simulink model "steer_by_wire"  (R2019b)
settings: Solver=FixedStepDiscrete  StartTime=0.0  StopTime=inf  RelTol=1e-3  EnableMultiTasking=on
undefined symbols (not defined in the file): DiscIntNeverNeededParam
settings Model: SimulationMode=external  Creator=guest  LastModifiedBy=cernylu6
settings DataIOCC: ReturnWorkspaceOutputs=off
settings OptimizationCC: PassReuseOutputArgsAs=Individual arguments  EfficientTunableParamExpr=on
settings DebuggingCC: ParameterTunabilityLossMsg=error  ArithmeticOperatorsInVariantConditions=warning
settings SFSimCC: SimUseLocalCustomCode=off  MATLABDynamicMemAlloc=off  CustomCodeUndefinedFunction=UseInterfaceOnly
settings RTWCC: Description=Linux Embedded Coder  SystemTargetFile=ert_linux.tlc  MakeCommand="make_rtw OPT_OPTS=\"-O2 -ggdb -Wall\" CC=arm-linux-gnueabihf-gcc CPP=arm-linux-gnueabihf-gcc"  TemplateMakefile=ert_linux.tmf  GenerateReport=on  RTWUseLocalCustomCode=off  IncludeHyperlinkInReport=on  LaunchReport=on  GenerateTraceInfo=on  GenerateTraceReport=on  GenerateTraceReportSl=on  GenerateTraceReportSf=on  GenerateTraceReportEml=on
settings CodeAppCC: ForceParamTrailComments=on  IgnoreCustomStorageClasses=off  OperatorAnnotations=on  SimulinkDataObjDesc=on  SFDataObjDesc=on  MATLABFcnDesc=on  InsertBlockDesc=on  StateflowObjectComments=on  MATLABSourceComments=on
settings STFCustomTargetCC: TargetLangStandard=C99 (ISO)  MultiwordLength=256  ModelReferenceCompliant=off  CombineOutputUpdateFcns=on  ERTCustomFileBanners=on  SupportContinuousTime=off  RemoveResetFunc=on  MATLABClassNameForMDSCustomization=Simulink.SoftwareTarget.ERTCustomization  SystemTargetFile=ert_linux.tlc
settings ERTTargetCC: TargetLangStandard=C99 (ISO)  ModelReferenceCompliant=off  ParMdlRefBuildCompliant=off  CompOptLevelCompliant=off  ConcurrentExecutionCompliant=off  SupportNonInlinedSFcns=on  ModelStepFunctionPrototypeControlCompliant=off  CPPClassGenCompliant=off  UseToolchainInfoCompliant=off  ExtMode=on  ExtModeMexArgs='192.168.136.74'  ERTCustomFileTemplate=ert_linux_file_process.tlc

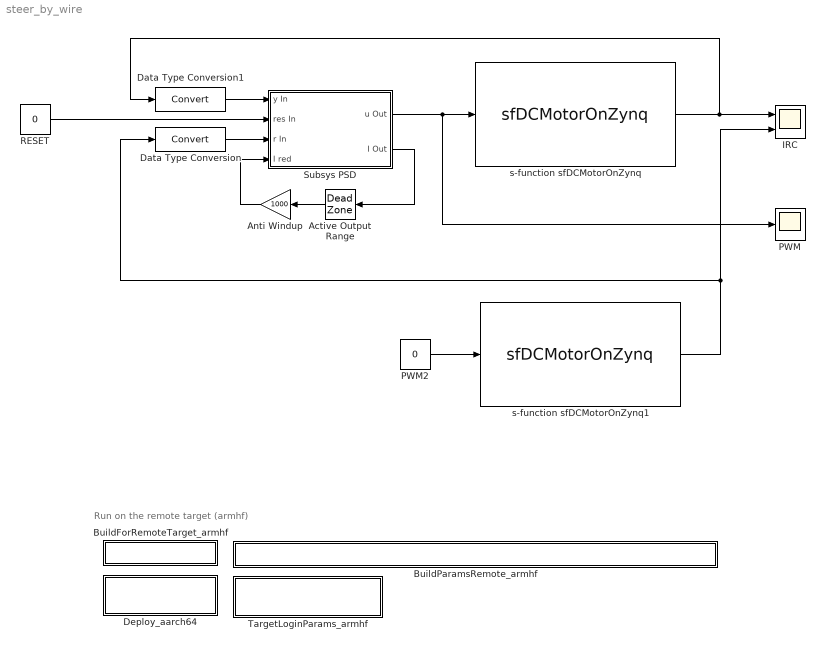
== system steer_by_wire ==
  note: Run on the remote target (armhf)
  "  RESET" : Constant  Value=0
      settings: OpenFcn=if get_param(gcbh,'value')=='0' set_param(gcbh,'value','1'); else set_param(gcbh,'value','0'); end;
  Active Output Range : DeadZone  LowerValue=-1  UpperValue=1  LinearizeAsGain=off
  Anti Windup : Gain  Gain=1000
  BuildForRemoteTarget_armhf : Subsystem
      settings: OpenFcn=ert_linux_build(gcs, 'BuildParamsRemote_armhf')
      mask Display: disp('Build')
  BuildParamsRemote_armhf : Subsystem  mask{make_command='make_rtw OPT_OPTS="-O2 -ggdb -Wall" CC=arm-linux-gnueabihf-gcc CPP=arm-linux-gnueabihf-gcc'}
      mask prompts: make_command "MakeCommand"
      mask Display: disp(get_param(gcb, 'make_command'));
  Data Type Conversion : DataTypeConversion
  Data Type Conversion1 : DataTypeConversion
  Deploy_aarch64 : Subsystem
      settings: OpenFcn=ert_linux_deploy_and_connect(gcs, 'TargetLoginParams_armhf');
      mask Display: disp('Deploy and\nconnect')
  IRC : Scope  NumInputPorts=2
  PWM : Scope
  PWM2 : Constant  Value=0
  Subsys PSD : Subsystem  mask(optimized PSD controller){P=0.01, I=0.1, D=0.0001, Ts=0.001}
      mask prompts: P "P proportional (P):"; I "I integral (I):"; D "D derivative (D):"; Ts "Sampling period (Ts):"
      mask help:
      | Type: Subsystem block.
      |
      | Description:
      |   Subsystem covers optimized PSD controller (PSD represents discretized PID).
      |
      | Requirements:
      |   Sampling period Ts.
      mask Help:
      | <b>Type:</b> Subsystem block.
      | <br><br>
      | <b>Description:</b><br>
      |   Subsystem covers optimized PSD controller (PSD represents discretized PID).
      | <br><br>
      | <b>Requirements:</b><br>
      |   Sampling period Ts.
      mask Display:
      | color('orange');disp('\n          Opt. PSD\n          Controller');
      | color('green');port_label('input', 1, 'w');
      | color('red');port_label('input', 2, ' RSTs');
      | color('lightblue');port_label('input', 3, 'r');
      | color('orange');port_label('input', 4, 'red I');
      | color('orange');port_label('output', 1, 'u ');
      | color('orange');port_label('output', 2, 'I  ');
      | color('red');disp('\n\n\n\n\n\n\n       P');
  TargetLoginParams_armhf : Subsystem  mask{trgt_ip_addr='192.168.136.74', trgt_username='root'}
      mask prompts: trgt_ip_addr "Target IP address"; trgt_username "Target username"
      mask Display:
      | ip_addr = get_param(gcb, 'trgt_ip_addr');
      | user = get_param(gcb, 'trgt_username');
      | 
      | fprintf('IP addr:\t %s\n User:\t %s ', ip_addr, user);
  s-function sfDCMotorOnZynq : S-Function  FunctionName=sfDCMotorOnZynq  Parameters=Ts,MOT_ID  SFunctionDeploymentMode=off  EnableBusSupport=off  mask{Ts=0.001, MOT_ID=0}
      mask prompts: Ts "Sampling period (Ts):"; MOT_ID "Motor ID:"
      mask help:
      | Input PWM is real number from interval [-1, 1].
      | Output IRC_POS is integer value.
      mask Display:
      | fprintf('MZ_APO DC Motor\ns-function\n(PMOD%d)\n', get_param(gcb, 'MOT_ID')-48);
      | port_label('input', 1, 'PWM')
      | port_label('output',1,'IRC_POS')
  s-function sfDCMotorOnZynq1 : S-Function  FunctionName=sfDCMotorOnZynq  Parameters=Ts,MOT_ID  SFunctionDeploymentMode=off  EnableBusSupport=off  mask{Ts=0.001, MOT_ID=1}
      mask prompts: Ts "Sampling period (Ts):"; MOT_ID "Motor ID:"
      mask help:
      | Input PWM is real number from interval [-1, 1].
      | Output IRC_POS is integer value.
      mask Display:
      | fprintf('MZ_APO DC Motor\ns-function\n(PMOD%d)\n', get_param(gcb, 'MOT_ID')-48);
      | port_label('input', 1, 'PWM')
      | port_label('output',1,'IRC_POS')
  wires:
  s-function sfDCMotorOnZynq/1 -> Data Type Conversion1/1, IRC/1
  PWM2/1 -> s-function sfDCMotorOnZynq1/1
  Subsys PSD/1(u Out) -> PWM/1, s-function sfDCMotorOnZynq/1
  s-function sfDCMotorOnZynq1/1 -> Data Type Conversion/1, IRC/2
  Active Output Range/1 -> Anti Windup/1
  Subsys PSD/2(I Out) -> Active Output Range/1
  Anti Windup/1 -> Subsys PSD/4(I red)
  Data Type Conversion1/1 -> Subsys PSD/1(y In)
  Data Type Conversion/1 -> Subsys PSD/3(r In)
  "  RESET"/1 -> Subsys PSD/2(res In)

== system steer_by_wire/BuildForRemoteTarget_armhf ==

== system steer_by_wire/BuildParamsRemote_armhf ==

== system steer_by_wire/Deploy_aarch64 ==

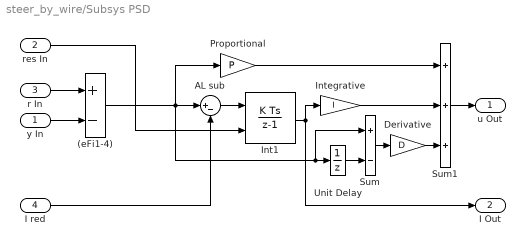
== system steer_by_wire/Subsys PSD ==
  y In : Inport  SampleTime=Ts
  res In : Inport  Port=2
  r In : Inport  Port=3  SampleTime=Ts
  I red : Inport  Port=4
  "  Derivative" : Gain  Gain=D  SaturateOnIntegerOverflow=on  OutDataTypeStr=Inherit: Same as input  ParamDataTypeStr=Inherit: Same as input
  (eFi1-4) : Sum  Inputs=+-  SaturateOnIntegerOverflow=on  InputSameDT=on  OutDataTypeStr=Inherit: Same as first input
  AL sub : Sum  Inputs=|+-  SaturateOnIntegerOverflow=on  InputSameDT=on  OutDataTypeStr=Inherit: Same as first input
  Int1 : DiscreteIntegrator  ExternalReset=level  SampleTime=-1  ICPrevOutput=DiscIntNeverNeededParam  ICPrevScaledInput=DiscIntNeverNeededParam
  Integrative : Gain  Gain=I  SaturateOnIntegerOverflow=on  OutDataTypeStr=Inherit: Same as input  ParamDataTypeStr=Inherit: Same as input
  Proportional : Gain  Gain=P  SaturateOnIntegerOverflow=on  OutDataTypeStr=Inherit: Same as input  ParamDataTypeStr=Inherit: Same as input
  Sum : Sum  Inputs=+-  SaturateOnIntegerOverflow=on  InputSameDT=on  OutDataTypeStr=Inherit: Same as first input
  Sum1 : Sum  Inputs=+++  SaturateOnIntegerOverflow=on  InputSameDT=on  OutDataTypeStr=Inherit: Same as first input
  Unit Delay : UnitDelay  SampleTime=Ts  HasFrameUpgradeWarning=on
  u Out : Outport
  I Out : Outport  Port=2
  wires:
  r In/1 -> (eFi1-4)/1
  y In/1 -> (eFi1-4)/2
  (eFi1-4)/1 -> Proportional/1, AL sub/1, Sum/1, Unit Delay/1
  "  Derivative"/1 -> Sum1/3
  Int1/1 -> I Out/1, Integrative/1
  Proportional/1 -> Sum1/1
  Sum1/1 -> u Out/1
  Sum/1 -> "  Derivative"/1
  Unit Delay/1 -> Sum/2
  res In/1 -> Int1/2
  AL sub/1 -> Int1/1
  I red/1 -> AL sub/2
  Integrative/1 -> Sum1/2

== system steer_by_wire/TargetLoginParams_armhf ==
